simulink model "DELETE_TEST"  (R2022a)
settings: Solver=VariableStepAuto  StartTime=0.0  StopTime=10.0  RelTol=1e-3
settings Model: Creator=user  LastModifiedBy=user

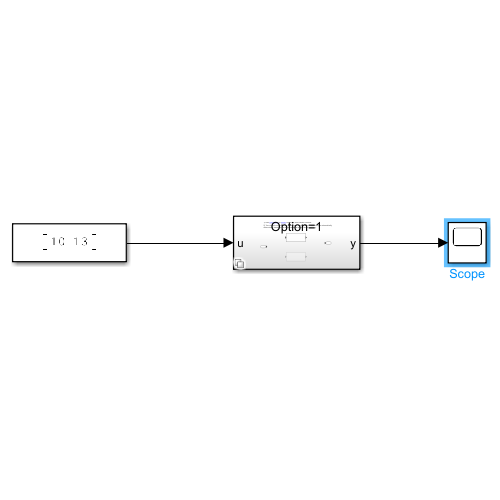
[thumbnail: Simulink's stored preview of the top-level diagram]
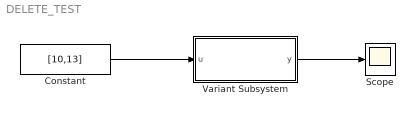
== system DELETE_TEST ==
  Constant : Constant  Value=[10,13]
  Scope : Scope
  Variant Subsystem : Subsystem  Variant=on
  wires:
  Constant/1 -> Variant Subsystem/1(u)
  Variant Subsystem/1(y) -> Scope/1

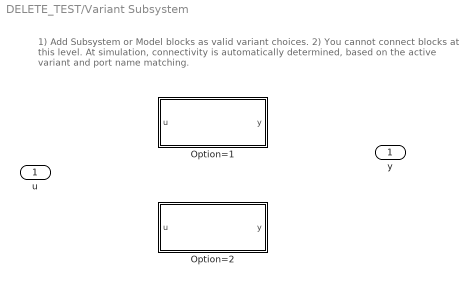
== system DELETE_TEST/Variant Subsystem ==
  note: 1) Add Subsystem or Model blocks as valid variant choices.
      | 2) You cannot connect blocks at this level. At simulation, connectivity is automatically
      | determined, based on the active variant and port name matching.
  u : Inport
  Option=1 : Subsystem  VariantControl=option==1
  Option=2 : Subsystem  VariantControl=option==2
  y : Outport

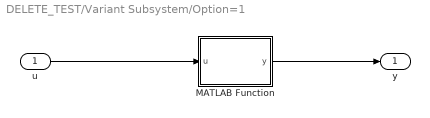
== system DELETE_TEST/Variant Subsystem/Option=1 ==
  u : Inport
  MATLAB Function : MATLAB Function  TreatAsAtomicUnit=on
  y : Outport
  wires:
  u/1 -> MATLAB Function/1(u)
  MATLAB Function/1(y) -> y/1

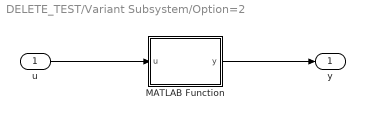
== system DELETE_TEST/Variant Subsystem/Option=2 ==
  u : Inport
  MATLAB Function : MATLAB Function  TreatAsAtomicUnit=on
  y : Outport
  wires:
  MATLAB Function/1(y) -> y/1
  u/1 -> MATLAB Function/1(u)

== matlab function DELETE_TEST/Variant Subsystem/Option=1/MATLAB Function ==
  data: u input; y output
function y = fcn(u)
y = u(2);

== matlab function DELETE_TEST/Variant Subsystem/Option=2/MATLAB Function ==
  data: u input; y output
function y = fcn(u)

y = -u;
